simulink model "L4_SIM"  (R2018a)
settings: Solver=ode1  StartTime=0.0  StopTime=60  FixedStep=GLB_FIXED_STEP_SIZE_CPV  RelTol=1e-3  EnableMultiTasking=on
undefined symbols (not defined in the file or in its folder): Cf, Chassis, Cr, CYCLE_ACC1_2A__AdaptiveCruiseCtrlMode, CYCLE_ACC1_2A__AdaptiveCruiseCtrlSetSpeed, CYCLE_CCVS1_00__CruiseCtrlSetSpeed, CYCLE_CCVS1_00__WheelBasedVehicleSpeed, CYCLE_EEC1_00__EngSpeed, CYCLE_ETC1_00__TransDrivelineEngaged, CYCLE_ETC2_00__TransActualGearRatio, CYCLE_ETC7_03__TransMode1Indicator, CYCLE_GPS_Latitude, CYCLE_GPS_Longitude, CYCLE_LFE1_00__EngFuelRate, CYCLE_Net_Engine_Percent_Torque, CYCLE_SSI2_03__PitchAngleExRange, CYCLE_TIME, CYCLE_UTM_Origin_X, CYCLE_UTM_Origin_Y, CYCLE_Vehicle_Distance, DiscIntNeverNeededParam, ENUM_J1939_PCC_STATE_T, ENUM_J1939_SWITCH_T, ENUM_STEERING_WHEEL_ANGLE_SENSOR_TYPE_T, GLB_FIXED_STEP_SIZE_CPV, GLB_TRANS_LOSS_TRQ_GEAR_STEP_MPV, GLB_TRANS_LOSS_TRQ_SPD_STEP_MPV, GLB_TRANS_LOSS_TRQ_TABLE_DATA_MPV, GLB_TRANS_LOSS_TRQ_TRQ_STEP_MPV, GLB_VEHICLE_CONFIG_ACCEL_PED_GATEWAY_APV, heading_0, Iz, L4_Controller, lf, lr, position_0, ptc_matlab_lib, STEERCTRL_10ms, SUB_ECU_L4_MABX, SUB_L4_Task_10ms, SUB_L4_Task_10ms_SUB_STEERCTRL, SUB_PLANT_Chassis, Task_10ms, Vx_0
libraries: EmE_MBD_Blockset x81, PTC_MBDS_LIB x71, simulink x38, simulink_extras x1, SUB_L4_Task_10000ms x1, SUB_L4_Task_1000ms x1, SUB_L4_Task_100ms x1, SUB_L4_Task_10ms_SUB_APTC x1, SUB_L4_Task_10ms_SUB_BRKPEDARB x1, SUB_L4_Task_10ms_SUB_FAULT_MANAGER x1, SUB_L4_Task_10ms_SUB_STATE_CONTROL x1, simulink_need_slupdate x1
(part 1 of 6)
settings Model: PauseTimes=1555  Creator=Sundeep.Tuteja  LastModifiedBy=Gennaro.Kukonu
settings SolverCC: AutoInsertRateTranBlk=on
settings OptimizationCC: DefaultUnderspecifiedDataType=single  LifeSpan=inf
settings DebuggingCC: SignalRangeChecking=error  AlgebraicLoopMsg=error  BlockPriorityViolationMsg=error  MinStepSizeMsg=error  TasksWithSamePriorityMsg=error  ParameterDowncastMsg=warning  UnderSpecifiedDataTypeMsg=warning  UnnecessaryDatatypeConvMsg=warning  SignalLabelMismatchMsg=warning  UnconnectedInputMsg=error  UniqueDataStoreMsg=error  BusObjectLabelMismatch=error  StateNameClashWarn=warning  SFExecutionAtInitializationDiag=none
settings CodeAppCC: StateflowObjectComments=on

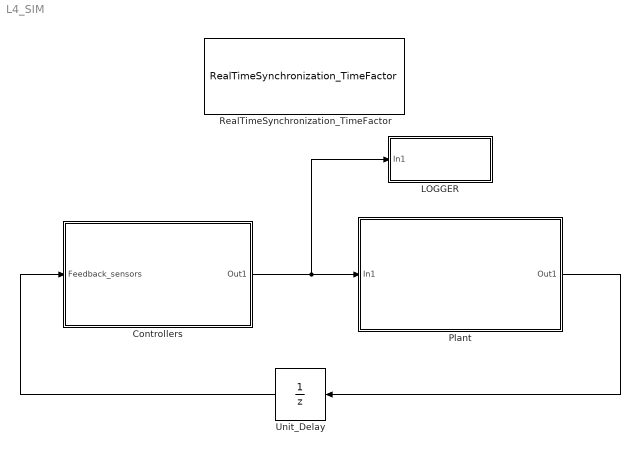
== system L4_SIM ==
  Controllers : Subsystem
  LOGGER : Subsystem
  Plant : Subsystem
      mask Display: image(fullfile(fileparts(which(bdroot(gcs))), '..', 'images', 'truckicon.jpg'));
  RealTimeSynchronization_TimeFactor : PTC_MBDS_LIB/Extras/HMI/RealTimeSynchronization_TimeFactor  Enable=off  TimeFactor=1  TimeFactor_prev=1  PTC_MBDS_BlockVersion=5.41  PTC_BlockType=PTC_MBDS_RealTimeSynchronization_TimeFactor
      settings: SourceProductName=PACCAR Technical Center MBDS Library
  Unit_Delay : UnitDelay  SampleTime=-1
      settings: AttributesFormatString=Init = %<InitialCondition>
  wires:
  Controllers/1(Out1) -> LOGGER/1(In1), Plant/1(In1)
  Plant/1(Out1) -> Unit_Delay/1
  Unit_Delay/1 -> Controllers/1(Feedback_sensors)

== system L4_SIM/Controllers ==
  Feedback_sensors : Inport
  Bus Creator : BusCreator  Inputs=5
  Drive_Cycle : Subsystem
  Operator : Subsystem
  Virtual_Controllers : Subsystem
  Out1 : Outport
  wires:
  Feedback_sensors/1 -> Drive_Cycle/1(Feedback_in)  "Feedback_sensors"
  Drive_Cycle/1(Cycle_out) -> Operator/1(Cycle_in)
  Drive_Cycle/2(Feedback_sensors_out) -> Operator/2(Feedback_sensors_in)
  Operator/1(Cycle_out) -> Virtual_Controllers/1(Cycle_in)
  Operator/2(Feedback_sensors_out) -> Virtual_Controllers/2(Feedback_sensors_in)
  Operator/3(Operator_out) -> Virtual_Controllers/3(Operator_in)
  Virtual_Controllers/1(Cycle_out) -> Bus Creator/1  "Cycle"
  Virtual_Controllers/2(Feedback_sensors_out) -> Bus Creator/2  "Feedback"
  Virtual_Controllers/3(Operator_out) -> Bus Creator/3  "Operator"
  Virtual_Controllers/4(Controller_out) -> Bus Creator/4  "Controller"
  Bus Creator/1 -> Out1/1
  Virtual_Controllers/5(Interfaces_out) -> Bus Creator/5  "Interface"

== system L4_SIM/LOGGER ==
  In1 : Inport
  Bus Creator : BusCreator  Inputs=14
  Bus Creator1 : BusCreator  Inputs=12
  Bus Selector : BusSelector  OutputSignals=Interface.CAN.EEC1_00.SPN513_ActualEngPercTorque,Interface.CAN.EEC1_00.SPN190_EngineSpeed,Interface.CAN.ETC2_00.SPN526_TransActualGearRatio,Interface.CAN.ETC2_00.SPN523_TransCurrentGear,Interface.CAN.EEC3_00.SPN514_NominalFrictionPercTorque,Interface.CAN.CCVS1_00.SPN84_WheelBasedVehicleSpeed,Interface.CAN.CCVS1_00.SPN86_CruiseControlSetSpeed,Interface.CAN.CCVS1_00.SPN527_CruiseControlState,Interface.CAN.EEC2_00.SPN91_AccelPedalPosition1,Interface.CAN.ERC1_0F.SPN520_ActualRetarderPercentTorque,Interface.CAN.ETC1_03.SPN560_TransDrivelineEngaged,Interface.CAN.SSI2_03.SPN4976_PitchAngleExtendedRange,Interface.CAN.CCVS3_00.SPN7319_CruiseControlSpeed,Interface.CAN.VDHR_31.SPN917_TotalVehicleDistanceHiResolution
  Bus Selector1 : BusSelector  OutputSignals=Controller
  Bus Selector2 : BusSelector  OutputSignals=AMT.ShiftControl.Internal.GearNumberCommand,AMT.ShiftControl.Internal.MainClutch,AMT.ShiftControl.Internal.ShiftControlState,AMT.ShiftControl.External.GearNumberActual,AMT.ShiftControl.External.TransStateLock,AMT.ShiftControl.External.TSC1_P32_TE.OCME,AMT.ShiftControl.External.TSC1_P32_TE.TrqReqE,PCI.EngTrqDemand,PCI.EngSpeedRPM,PCI.DriverDemPercentTrq,ABS.FrontAxleSpd,L4_MABX.10msTask.APTC.APTC_arb_pedal_position
  SignalConversion{,1..25} (26 alike) : SignalConversion  ConversionOutput=Contiguous copy  OverrideOpt=off
  Terminator : Terminator
      settings: InitFcn=|
      | try
      |    MBDS_BlockCallback('Update', gcb);
      | end
  Terminator1 : Terminator
      settings: InitFcn=|
      | try
      |    MBDS_BlockCallback('Update', gcb);
      | end
  wires:
  In1/1 -> Bus Selector1/1, Bus Selector/1
  Bus Creator/1 -> Terminator/1
  Bus Selector1/1 -> Bus Selector2/1  "<Controller>"
  Bus Creator1/1 -> Terminator1/1
  Bus Selector/1 -> SignalConversion/1  "<SPN513_ActualEngPercTorque>"
  SignalConversion/1 -> Bus Creator/1  "SPN513_ActualEngPercTorque"
  Bus Selector/2 -> SignalConversion1/1  "<SPN190_EngineSpeed>"
  SignalConversion1/1 -> Bus Creator/2  "SPN190_EngineSpeed"
  Bus Selector/3 -> SignalConversion2/1  "<SPN526_TransActualGearRatio>"
  SignalConversion2/1 -> Bus Creator/3  "SPN526_TransActualGearRatio"
  Bus Selector/4 -> SignalConversion3/1  "<SPN523_TransCurrentGear>"
  SignalConversion3/1 -> Bus Creator/4  "SPN523_TransCurrentGear"
  Bus Selector/5 -> SignalConversion4/1  "<SPN514_NominalFrictionPercTorque>"
  SignalConversion4/1 -> Bus Creator/5  "SPN514_NominalFrictionPercTorque"
  Bus Selector/6 -> SignalConversion5/1  "<SPN84_WheelBasedVehicleSpeed>"
  SignalConversion5/1 -> Bus Creator/6  "SPN84_WheelBasedVehicleSpeed"
  Bus Selector/7 -> SignalConversion6/1  "<SPN86_CruiseControlSetSpeed>"
  SignalConversion6/1 -> Bus Creator/7  "SPN86_CruiseControlSetSpeed"
  Bus Selector/8 -> SignalConversion7/1  "<SPN527_CruiseControlState>"
  SignalConversion7/1 -> Bus Creator/8  "SPN527_CruiseControlState"
  Bus Selector/9 -> SignalConversion8/1  "<SPN91_AccelPedalPosition1>"
  SignalConversion8/1 -> Bus Creator/9  "SPN91_AccelPedalPosition1"
  Bus Selector/10 -> SignalConversion9/1  "<SPN520_ActualRetarderPercentTorque>"
  SignalConversion9/1 -> Bus Creator/10  "SPN520_ActualRetarderPercentTorque"
  Bus Selector/11 -> SignalConversion10/1  "<SPN560_TransDrivelineEngaged>"
  SignalConversion10/1 -> Bus Creator/11  "SPN560_TransDrivelineEngaged"
  Bus Selector/12 -> SignalConversion11/1  "<SPN4976_PitchAngleExtendedRange>"
  SignalConversion11/1 -> Bus Creator/12  "SPN4976_PitchAngleExtendedRange"
  Bus Selector/13 -> SignalConversion12/1  "<SPN7319_CruiseControlSpeed>"
  SignalConversion12/1 -> Bus Creator/13  "SPN7319_CruiseControlSpeed"
  Bus Selector/14 -> SignalConversion13/1  "<SPN917_TotalVehicleDistanceHiResolution>"
  SignalConversion13/1 -> Bus Creator/14  "SPN917_TotalVehicleDistanceHiResolution"
  Bus Selector2/11 -> SignalConversion14/1  "<FrontAxleSpd>"
  SignalConversion14/1 -> Bus Creator1/11  "FrontAxleSpd"
  Bus Selector2/10 -> SignalConversion15/1  "<DriverDemPercentTrq>"
  SignalConversion15/1 -> Bus Creator1/10  "DriverDemPercentTrq"
  Bus Selector2/9 -> SignalConversion16/1  "<EngSpeedRPM>"
  SignalConversion16/1 -> Bus Creator1/9  "EngSpeedRPM"
  Bus Selector2/8 -> SignalConversion17/1  "<EngTrqDemand>"
  SignalConversion17/1 -> Bus Creator1/8  "EngTrqDemand"
  Bus Selector2/7 -> SignalConversion18/1  "<TrqReqE>"
  SignalConversion18/1 -> Bus Creator1/7  "TrqReq"
  Bus Selector2/6 -> SignalConversion19/1  "<OCME>"
  SignalConversion19/1 -> Bus Creator1/6  "OCM"
  Bus Selector2/5 -> SignalConversion20/1  "<TransStateLock>"
  SignalConversion20/1 -> Bus Creator1/5  "TransStateLock"
  Bus Selector2/4 -> SignalConversion21/1  "<GearNumberActual>"
  SignalConversion21/1 -> Bus Creator1/4  "GearNumberActual"
  Bus Selector2/3 -> SignalConversion22/1  "<ShiftControlState>"
  SignalConversion22/1 -> Bus Creator1/3  "ShiftControlState"
  Bus Selector2/2 -> SignalConversion23/1  "<MainClutch>"
  SignalConversion23/1 -> Bus Creator1/2  "MainClutch"
  Bus Selector2/1 -> SignalConversion24/1  "<GearNumberCommand>"
  SignalConversion24/1 -> Bus Creator1/1  "GearNumberCommand"
  Bus Selector2/12 -> SignalConversion25/1  "<APTC_arb_pedal_position>"
  SignalConversion25/1 -> Bus Creator1/12  "AcceleratorPedalPosOut"

== system L4_SIM/Plant ==
  In1 : Inport
  Bus Creator : BusCreator  Inputs=3
  Bus Selector : BusSelector  OutputSignals=Feedback,Operator,Cycle,Controller
  PlantModel : Subsystem
  Out1 : Outport
  wires:
  In1/1 -> Bus Selector/1
  Bus Selector/3 -> PlantModel/3(Cycle)  "<Cycle>"
  Bus Selector/2 -> PlantModel/2(Driver)  "<Operator>"
  Bus Selector/4 -> PlantModel/4(Control)  "<Controller>"
  PlantModel/2(Engine_O) -> Bus Creator/2  "Engine"
  PlantModel/1(Chassis_O) -> Bus Creator/1  "Chassis"
  Bus Creator/1 -> Out1/1
  Bus Selector/1 -> PlantModel/1(FB)  "<Feedback>"
  PlantModel/3(Nav_O) -> Bus Creator/3  "Navigation"

== system L4_SIM/Controllers/Drive_Cycle ==
  Feedback_in : Inport
  Bias : Bias  Bias=-1
  Bus Selector1 : BusSelector  OutputSignals=ActualVehicleDistance
  Bus Selector2 : BusSelector  OutputSignals=Chassis.MeasuredVehicleSpeed_kph
  Constant1 : PTC_MBDS_LIB/Extras/Sources/Constant  Value2=1/3.6  PTC_MBDS_BlockVersion=5.41  PTC_BlockType=PTC_MBDS_Constant
      settings: SourceProductName=PACCAR Technical Center MBDS Library
  Constant3 : PTC_MBDS_LIB/Extras/Sources/Constant  Value2=CYCLE_Vehicle_Distance  PTC_MBDS_BlockVersion=5.41  PTC_BlockType=PTC_MBDS_Constant
      settings: SourceProductName=PACCAR Technical Center MBDS Library
      settings: AttributesFormatString=|
      | Value: <16520 X 1>
      | Unit: 'm'
  DriveCycle : Subsystem
  GE : PTC_MBDS_LIB/MBDS Standard Library/Basic Operations/Logic and Bit Operations/GE  InputSameDT=on  PTC_MBDS_BlockVersion=5.41  PTC_BlockType=PTC_MBDS_GE
      settings: SourceProductName=PACCAR Technical Center MBDS Library
  Product : Product  Inputs=**  OutDataTypeStr=Inherit: Inherit via back propagation  SaturateOnIntegerOverflow=on  InputSameDT=on
      settings: AttributesFormatString=Saturate: %<SaturateOnIntegerOverflow>
  Selector2 : Selector  IndexOptions=Index vector (port)  Indices=[1 3]  OutputSizes=1
  Stop Simulation : Stop
  Width1 : Width  DataType=uint32
  Cycle_out : Outport
  Feedback_sensors_out : Outport  Port=2
  wires:
  Feedback_in/1 -> Feedback_sensors_out/1, Bus Selector2/1
  Constant1/1 -> Product/2
  Product/1 -> DriveCycle/1(MeasuredVehicleSpeed_mps)  "MeasuredVehicleSpeed_mps"
  Bus Selector2/1 -> Product/1  "<MeasuredVehicleSpeed_kph>"
  DriveCycle/1(Cycle_out) -> Bus Selector1/1, Cycle_out/1  "Cycle"
  Selector2/1 -> Bias/1
  Width1/1 -> Selector2/2
  Constant3/1 -> Selector2/1, Width1/1  "CYCLE_Vehicle_Distance"
  Bus Selector1/1 -> GE/1  "<ActualVehicleDistance>"
  GE/1 -> Stop Simulation/1
  Bias/1 -> GE/2

== system L4_SIM/Controllers/Operator ==
  Cycle_in : Inport
  Feedback_sensors_in : Inport  Port=2
  Bus Creator : BusCreator  Inputs=4
  Bus Selector : BusSelector  OutputSignals=RefVehSpeed,RefVehPosition,CCSetSpeed,L4OperatorEnable
  Bus Selector1 : BusSelector  OutputSignals=Chassis.MeasuredVehicleSpeed_kph,Navigation.VehPosition
  Subsystem : Subsystem
  Cycle_out : Outport
  Feedback_sensors_out : Outport  Port=2
  Operator_out : Outport  Port=3
  wires:
  Cycle_in/1 -> Cycle_out/1, Bus Selector/1  "Cycle"
  Feedback_sensors_in/1 -> Bus Selector1/1, Feedback_sensors_out/1  "Feedback_sensors"
  Bus Selector/1 -> Subsystem/1(RefVehSpeed[km/h])  "<RefVehSpeed>"
  Bus Selector/3 -> Subsystem/3(CCSetSpeed[km/h])  "<CCSetSpeed>"
  Bus Selector1/1 -> Subsystem/5(MeasuredVehicleSpeed[km/h])  "<MeasuredVehicleSpeed_kph>"
  Subsystem/1(BrkDrv[0-1]) -> Bus Creator/1
  Subsystem/2(PedDrv[0-1]) -> Bus Creator/2
  Bus Creator/1 -> Operator_out/1  "Operator"
  Subsystem/3(OperatorEnable) -> Bus Creator/3  "OperatorEnable"
  Bus Selector/4 -> Subsystem/4(OperatorEnableCycle)  "<L4OperatorEnable>"
  Bus Selector/2 -> Subsystem/2(RefVehPosition[m])  "<RefVehPosition>"
  Subsystem/4(TargetHeading) -> Bus Creator/4  "TargetHeading"
  Bus Selector1/2 -> Subsystem/6(MeasuredVehiclePosition[m])  "<VehPosition>"

== system L4_SIM/Controllers/Virtual_Controllers ==
  Cycle_in : Inport
  Feedback_sensors_in : Inport  Port=2
  Operator_in : Inport  Port=3
  ABS : Subsystem
  Bus Creator1 : BusCreator  Inputs=4
  Bus Creator2 : BusCreator  Inputs=9
  ERAD : Subsystem
  Interface_Abstraction : Subsystem
  L4_MABX : Subsystem
  PACC : Subsystem
  PCC : Subsystem
  PCI : Subsystem
  TCM : Subsystem
  Unit_Delay : UnitDelay  SampleTime=-1
      settings: AttributesFormatString=Init = %<InitialCondition>
  VECU : Subsystem
  VEMC : Subsystem
  Cycle_out : Outport
  Feedback_sensors_out : Outport  Port=2
  Operator_out : Outport  Port=3
  Controller_out : Outport  Port=4
  Interfaces_out : Outport  Port=5
  wires:
  Bus Creator1/1 -> Interface_Abstraction/1(Inport)
  Interface_Abstraction/1(Outport) -> ERAD/1(In1), TCM/1(In1), VEMC/1(In1), VECU/1(In1), PCI/1(In), PCC/1(In1), PACC/1(In1), L4_MABX/1(input), Interfaces_out/1, ABS/1(input)
  Cycle_in/1 -> Cycle_out/1, Bus Creator1/1  "Cycle"
  Feedback_sensors_in/1 -> Bus Creator1/2, Feedback_sensors_out/1  "Feedback_sensors"
  Operator_in/1 -> Bus Creator1/3, Operator_out/1  "Operator"
  TCM/1(Out1) -> Bus Creator2/7  "AMT"
  ABS/1(Out1) -> Bus Creator2/1  "ABS"
  PCI/1(Out1) -> Bus Creator2/6  "PCI"
  PACC/1(Out1) -> Bus Creator2/4  "PACC"
  L4_MABX/1(Out1) -> Bus Creator2/3  "L4_MABX"
  PCC/1(Out1) -> Bus Creator2/5  "PCC"
  Bus Creator2/1 -> Unit_Delay/1, Controller_out/1  "Feedback_controllers"
  ERAD/1(Out1) -> Bus Creator2/2  "ERAD"
  Unit_Delay/1 -> Bus Creator1/4  "Feedback_controllers"
  VECU/1(Out1) -> Bus Creator2/8  "VECU"
  VEMC/1(Out1) -> Bus Creator2/9  "VEMC"

== system L4_SIM/Plant/PlantModel ==
  FB : Inport
  Driver : Inport  Port=2
  Cycle : Inport  Port=3
  Control : Inport  Port=4
  Bus Selector : BusSelector  OutputSignals=BrkDrv
  Bus Selector2 : BusSelector  OutputSignals=PCI,AMT,ABS,L4_MABX
  Chassis : Subsystem  AncestorBlock=SUB_PLANT_Chassis/Chassis
  Engine : SUB_PLANT_Engine/Engine
      link override Bus Selector1: OutputSignals=Chassis.TrqFromClutch,Chassis.ClutchState,Chassis.EngSpdClutchClosed
  Navigation : Subsystem
  Chassis_O : Outport
  Engine_O : Outport  Port=2
  Nav_O : Outport  Port=3
  wires:
  Engine/1 -> Chassis/1(Engine), Engine_O/1
  Driver/1 -> Bus Selector/1
  Bus Selector/1 -> Chassis/2(FoundationBrakes)  "<BrkDrv>"
  Cycle/1 -> Chassis/4(Cycle)
  Control/1 -> Bus Selector2/1
  Bus Selector2/1 -> Engine/2  "<PCI>"
  Bus Selector2/2 -> Chassis/3(AMT)  "<AMT>"
  Bus Selector2/3 -> Chassis/5(ABS)  "<ABS>"
  Chassis/1(ChassisMdl_O) -> Navigation/1(In1), Chassis_O/1
  Bus Selector2/4 -> Chassis/6(L4_MABX)  "<L4_MABX>"
  FB/1 -> Chassis/7(Navigation), Engine/1
  Navigation/1(Out1) -> Nav_O/1  "Navigation"

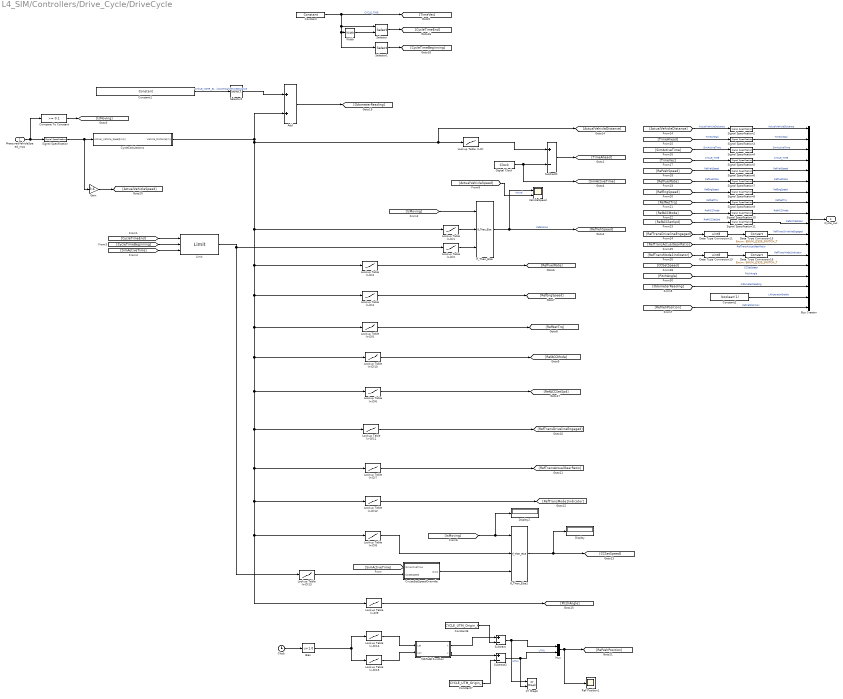
== system L4_SIM/Controllers/Drive_Cycle/DriveCycle ==
  MeasuredVehicleSpeed_mps : Inport
  Add : Sum  OutDataTypeStr=Inherit: Inherit via back propagation  SaturateOnIntegerOverflow=on  InputSameDT=on
      settings: AttributesFormatString=Saturate: %<SaturateOnIntegerOverflow>
  Bias : Bias  Bias=1.0
  Bus Creator : BusCreator  Inputs=18
  Clock : Clock
  Compare To Constant : simulink/Logic and Bit Operations/Compare To Constant  relop=>=  const=0.1  OutDataTypeStr=boolean
  Constant : PTC_MBDS_LIB/Extras/Sources/Constant  Value2=CYCLE_TIME  PTC_MBDS_BlockVersion=5.41  PTC_BlockType=PTC_MBDS_Constant
      settings: SourceProductName=PACCAR Technical Center MBDS Library
      settings: AttributesFormatString=|
      | Value: <16520 X 1>
      | Unit: 's'
  Constant1 : PTC_MBDS_LIB/Extras/Sources/Constant  Value2=CYCLE_VDHR_31__HghRslutionTotalVehicleDistance  PTC_MBDS_BlockVersion=5.41  PTC_BlockType=PTC_MBDS_Constant
      settings: SourceProductName=PACCAR Technical Center MBDS Library
      settings: AttributesFormatString=|
      | Value: <16520 X 1>
      | Unit: 'm'
  Constant2 : Constant  Value=boolean(1)
  Constant6 : Constant  Value=CYCLE_UTM_Origin_X
  Constant7 : Constant  Value=CYCLE_UTM_Origin_Y
  CruiseSetSpeedOverride : Subsystem
  CycleCalculations : Subsystem
  Data Type Conversion11 : DataTypeConversion  OutDataTypeStr=uint8  SaturateOnIntegerOverflow=on
  Data Type Conversion13 : DataTypeConversion  OutDataTypeStr=uint8  SaturateOnIntegerOverflow=on
  Data Type Conversion15 : DataTypeConversion  OutDataTypeStr=Enum: ENUM_J1939_SWITCH_T  SaturateOnIntegerOverflow=on
  Data Type Conversion16 : DataTypeConversion  OutDataTypeStr=Enum: ENUM_J1939_SWITCH_T  SaturateOnIntegerOverflow=on
  Digital Clock : DigitalClock  SampleTime=GLB_FIXED_STEP_SIZE_CPV
  Display : Display
  Display2 : Display
  Gain : Gain  Gain=3.6
  If_Then_Else : PTC_MBDS_LIB/Extras/Signal Routing/If_Then_Else  PTC_MBDS_BlockVersion=5.41  PTC_BlockType=PTC_MBDS_If_Then_Else
      settings: SourceProductName=PACCAR Technical Center MBDS Library
  If_Then_Else1 : PTC_MBDS_LIB/Extras/Signal Routing/If_Then_Else  PTC_MBDS_BlockVersion=5.41  PTC_BlockType=PTC_MBDS_If_Then_Else
      settings: SourceProductName=PACCAR Technical Center MBDS Library
  Limit : PTC_MBDS_LIB/MBDS Standard Library/Basic Operations/Non-Linear Operations/Limit  MXMN_Enabled=on  MX=0  MN=0  B_min_Enabled=off  B_max_Enabled=off  OutDataTypeStr=Inherit: Inherit via back propagation  SaturateOnIntegerOverflow=on  InputSameDT=on  InOutSameDT=on  PTC_MBDS_BlockVersion=5.41  PTC_BlockType=PTC_MBDS_Limit
      settings: AttributesFormatString=Saturate: on  SourceProductName=PACCAR Technical Center MBDS Library
  Lookup Table (n-D) : Lookup_n-D  NumberOfTableDimensions=1  BreakpointsForDimension1=CYCLE_Vehicle_Distance  Table=CYCLE_TIME  ExtrapMethod=Clip  DiagnosticForOutOfRangeInput=Error  InputSameDT=on
  Lookup Table (n-D)1 : Lookup_n-D  NumberOfTableDimensions=1  BreakpointsForDimension1=CYCLE_Vehicle_Distance  Table=CYCLE_CCVS1_00__WheelBasedVehicleSpeed  ExtrapMethod=Clip  DiagnosticForOutOfRangeInput=Error  InputSameDT=on
  Lookup Table (n-D)10 : Lookup_n-D  NumberOfTableDimensions=1  BreakpointsForDimension1=CYCLE_Vehicle_Distance  Table=CYCLE_ACC1_2A__AdaptiveCruiseCtrlMode  InterpMethod=Flat  ExtrapMethod=Clip  DiagnosticForOutOfRangeInput=Error  InputSameDT=on
  Lookup Table (n-D)11 : Lookup_n-D  NumberOfTableDimensions=1  BreakpointsForDimension1=CYCLE_Vehicle_Distance  Table=CYCLE_ETC1_00__TransDrivelineEngaged  InterpMethod=Flat  ExtrapMethod=Clip  DiagnosticForOutOfRangeInput=Error  InputSameDT=on
  Lookup Table (n-D)12 : Lookup_n-D  NumberOfTableDimensions=1  BreakpointsForDimension1=CYCLE_Vehicle_Distance  Table=CYCLE_ETC7_03__TransMode1Indicator  InterpMethod=Flat  ExtrapMethod=Clip  DiagnosticForOutOfRangeInput=Error  InputSameDT=on
  Lookup Table (n-D)13 : Lookup_n-D  NumberOfTableDimensions=1  BreakpointsForDimension1=CYCLE_TIME  Table=CYCLE_CCVS1_00__CruiseCtrlSetSpeed  ExtrapMethod=Clip  DiagnosticForOutOfRangeInput=Error  InputSameDT=on
  Lookup Table (n-D)14 : Lookup_n-D  NumberOfTableDimensions=1  BreakpointsForDimension1=CYCLE_TIME  Table=CYCLE_GPS_Latitude  ExtrapMethod=Clip  DiagnosticForOutOfRangeInput=Error  InputSameDT=on
  Lookup Table (n-D)15 : Lookup_n-D  NumberOfTableDimensions=1  BreakpointsForDimension1=CYCLE_TIME  Table=CYCLE_GPS_Longitude  ExtrapMethod=Clip  DiagnosticForOutOfRangeInput=Error  InputSameDT=on
  Lookup Table (n-D)2 : Lookup_n-D  NumberOfTableDimensions=1  BreakpointsForDimension1=CYCLE_TIME  Table=CYCLE_CCVS1_00__WheelBasedVehicleSpeed  ExtrapMethod=Clip  DiagnosticForOutOfRangeInput=Error  InputSameDT=on
  Lookup Table (n-D)3 : Lookup_n-D  NumberOfTableDimensions=1  BreakpointsForDimension1=CYCLE_Vehicle_Distance  Table=CYCLE_LFE1_00__EngFuelRate  ExtrapMethod=Clip  DiagnosticForOutOfRangeInput=Error  InputSameDT=on
  Lookup Table (n-D)4 : Lookup_n-D  NumberOfTableDimensions=1  BreakpointsForDimension1=CYCLE_Vehicle_Distance  Table=CYCLE_EEC1_00__EngSpeed  ExtrapMethod=Clip  DiagnosticForOutOfRangeInput=Error  InputSameDT=on
  Lookup Table (n-D)5 : Lookup_n-D  NumberOfTableDimensions=1  BreakpointsForDimension1=CYCLE_Vehicle_Distance  Table=CYCLE_Net_Engine_Percent_Torque  ExtrapMethod=Clip  DiagnosticForOutOfRangeInput=Error  InputSameDT=on
  Lookup Table (n-D)6 : Lookup_n-D  NumberOfTableDimensions=1  BreakpointsForDimension1=CYCLE_Vehicle_Distance  Table=CYCLE_ACC1_2A__AdaptiveCruiseCtrlSetSpeed  ExtrapMethod=Clip  DiagnosticForOutOfRangeInput=Error  InputSameDT=on
  Lookup Table (n-D)7 : Lookup_n-D  NumberOfTableDimensions=1  BreakpointsForDimension1=CYCLE_Vehicle_Distance  Table=CYCLE_ETC2_00__TransActualGearRatio  ExtrapMethod=Clip  DiagnosticForOutOfRangeInput=Error  InputSameDT=on
  Lookup Table (n-D)8 : Lookup_n-D  NumberOfTableDimensions=1  BreakpointsForDimension1=CYCLE_Vehicle_Distance  Table=CYCLE_CCVS1_00__CruiseCtrlSetSpeed  ExtrapMethod=Clip  DiagnosticForOutOfRangeInput=Error  InputSameDT=on
  Lookup Table (n-D)9 : Lookup_n-D  NumberOfTableDimensions=1  BreakpointsForDimension1=CYCLE_Vehicle_Distance  Table=CYCLE_SSI2_03__PitchAngleExRange  ExtrapMethod=Clip  DiagnosticForOutOfRangeInput=Error  InputSameDT=on
  MATLAB Function : MATLAB Function  TreatAsAtomicUnit=on
  Mux : Mux  Inputs=2
  Ref Position1 : Scope
  Selector : Selector  IndexOptions=Index vector (port)  Indices=[1 3]  OutputSizes=1
  Selector1 : Selector  IndexOptions=Index vector (dialog)  Indices=1  OutputSizes=1
  Selector2 : Selector  IndexOptions=Index vector (dialog)  Indices=1  OutputSizes=1
  Signal Specification{,2..11} (11 alike) : SignalSpecification  OutDataTypeStr=double
  Subtract : Sum  Inputs=+-
  Subtract1 : Sum  Inputs=+-  OutDataTypeStr=Inherit: Inherit via back propagation  SaturateOnIntegerOverflow=on  InputSameDT=on
      settings: AttributesFormatString=Saturate: %<SaturateOnIntegerOverflow>
  Subtract2 : Sum  Inputs=+-
  VehicleSpeed : Scope  NumInputPorts=2
  Width : Width  DataType=uint32
  XY Graph : simulink/Sinks/XY Graph  xmin=-100  xmax=100  ymin=-100  ymax=100  st=-1
  Cycle_out : Outport
  wires:
  MeasuredVehicleSpeed_mps/1 -> Signal Specification/1, Compare To Constant/1
  Lookup Table (n-D)/1 -> Subtract1/1
  Digital Clock/1 -> [SimActiveTime], Subtract1/2
  Subtract1/1 -> [TimeAhead]
  Compare To Constant/1 -> [IsMoving]
  [IsMoving] -> If_Then_Else/1
  Lookup Table (n-D)2/1 -> If_Then_Else/3
  Lookup Table (n-D)3/1 -> [RefFuelRate]
  Lookup Table (n-D)5/1 -> [RefNetTrq]
  Lookup Table (n-D)10/1 -> [RefACCMode]
  [RefTransDrivelineEngaged] -> Data Type Conversion11/1
  [RefTransMode1Indicator] -> Data Type Conversion13/1
  Bus Creator/1 -> Cycle_out/1
  [ActualVehicleDistance] -> Signal Specification2/1  "ActualVehicleDistance"
  [TimeAhead] -> Signal Specification3/1  "TimeAhead"
  [SimActiveTime] -> Signal Specification4/1  "SimActiveTime"
  [TimeVec] -> Signal Specification5/1  "CYCLE_TIME"
  [RefVehSpeed] -> Signal Specification6/1  "RefVehSpeed"
  [RefFuelRate] -> Signal Specification7/1  "RefFuelRate"
  [RefEngSpeed] -> Signal Specification8/1  "RefEngSpeed"
  [RefNetTrq] -> Signal Specification9/1  "RefNetTrq"
  [RefACCSetSpd] -> Signal Specification11/1  "RefACCSetSpd"
  Data Type Conversion11/1 -> Data Type Conversion15/1
  Data Type Conversion13/1 -> Data Type Conversion16/1
  [RefACCMode] -> Signal Specification10/1  "RefACCMode"
  Lookup Table (n-D)1/1 -> If_Then_Else/2
  Lookup Table (n-D)4/1 -> [RefEngSpeed]
  Lookup Table (n-D)6/1 -> [RefACCSetSpd]
  Lookup Table (n-D)11/1 -> [RefTransDrivelineEngaged]
  Lookup Table (n-D)7/1 -> [RefTransActualGearRatio]
  Lookup Table (n-D)12/1 -> [RefTransMode1Indicator]
  Lookup Table (n-D)9/1 -> [PitchAngle]
  Lookup Table (n-D)8/1 -> If_Then_Else1/2
  [SimActiveTime] -> CruiseSetSpeedOverride/1(SimActiveTime)
  [SimActiveTime] -> Limit/3
  Constant/1 -> [TimeVec], Selector1/1, Width/1, Selector/1  "CYCLE_TIME"
  Width/1 -> Selector/2
  Selector/1 -> [CycleTimeEnd]
  [CycleTimeEnd] -> Limit/1
  Selector1/1 -> [CycleTimeBeginning]
  [CycleTimeBeginning] -> Limit/2
  Constant1/1 -> Selector2/1  "CYCLE_VDHR_31__HghRslutionTotalVehicleDistance"
  Add/1 -> [OdometerReading]
  Selector2/1 -> Add/1
  Data Type Conversion15/1 -> Bus Creator/11  "RefTransDrivelineEngaged"
  Data Type Conversion16/1 -> Bus Creator/13  "RefTransMode1Indicator"
  Signal Specification2/1 -> Bus Creator/1  "ActualVehicleDistance"
  Signal Specification3/1 -> Bus Creator/2  "TimeAhead"
  Signal Specification4/1 -> Bus Creator/3  "SimActiveTime"
  Signal Specification5/1 -> Bus Creator/4  "CYCLE_TIME"
  Signal Specification6/1 -> Bus Creator/5  "RefVehSpeed"
  Signal Specification7/1 -> Bus Creator/6  "RefFuelRate"
  Signal Specification8/1 -> Bus Creator/7  "RefEngSpeed"
  Signal Specification9/1 -> Bus Creator/8  "RefNetTrq"
  Signal Specification10/1 -> Bus Creator/9  "RefACCMode"
  Signal Specification11/1 -> Bus Creator/10  "RefACCSetSpd"
  [RefTransActualGearRatio] -> Bus Creator/12  "RefTransActualGearRatio"
  [CCSetSpeed] -> Bus Creator/14  "CCSetSpeed"
  [PitchAngle] -> Bus Creator/15  "PitchAngle"
  [OdometerReading] -> Bus Creator/16  "OdometerReading"
  Limit/1 -> Lookup Table (n-D)13/1, Lookup Table (n-D)2/1
  If_Then_Else1/1 -> Display/1, [CCSetSpeed]
  [IsMoving] -> Display2/1, If_Then_Else1/1
  CruiseSetSpeedOverride/1(Out1) -> If_Then_Else1/3
  Lookup Table (n-D)13/1 -> CruiseSetSpeedOverride/2(CCSetSpeed)
  Constant2/1 -> Bus Creator/17  "L4OperatorEnable"
  Constant6/1 -> Subtract/2
  CycleCalculations/1(Vehicle_Distance[m]) -> Lookup Table (n-D)/1, [ActualVehicleDistance], Lookup Table (n-D)9/1, Lookup Table (n-D)8/1, Lookup Table (n-D)12/1, Lookup Table (n-D)7/1, Lookup Table (n-D)11/1, Lookup Table (n-D)6/1, Lookup Table (n-D)10/1, Lookup Table (n-D)5/1, Lookup Table (n-D)4/1, Lookup Table (n-D)3/1, Lookup Table (n-D)1/1, Add/2
  MATLAB Function/1(x) -> Subtract/1
  Lookup Table (n-D)14/1 -> MATLAB Function/1(Lat)
  Lookup Table (n-D)15/1 -> MATLAB Function/2(Lon)
  MATLAB Function/2(y) -> Subtract2/1
  Constant7/1 -> Subtract2/2
  If_Then_Else/1 -> VehicleSpeed/1, [RefVehSpeed]  "Reference"
  [ActualVehicleSpeed] -> VehicleSpeed/2  "Actual"
  Signal Specification/1 -> Gain/1, CycleCalculations/1(Actual_Vehicle_Speed[m/s])
  Gain/1 -> [ActualVehicleSpeed]
  Subtract2/1 -> XY Graph/2, Mux/2  "UTMy"
  Subtract/1 -> XY Graph/1, Mux/1  "UTMx"
  Bias/1 -> Lookup Table (n-D)15/1, Lookup Table (n-D)14/1
  Clock/1 -> Bias/1
  Mux/1 -> Ref Position1/1, [RefVehPosition]
  [RefVehPosition] -> Bus Creator/18  "RefVehPosition"

== system L4_SIM/Controllers/Operator/Subsystem ==
  note: Gains Added in own block
      | so they can be changed in
      | ICR_init.m file.  Acc and Brk
      | Gains should be equal, or it
      | will cause dynamic issues (PID
      | for Acc and Brk are exactly the
      | same, making different gains
      | between the pedals will cause
      | the model to behave differently).
      | This is applicable for the dyno.
  RefVehSpeed[km/h] : Inport  Unit=km/h
  RefVehPosition[m] : Inport  Port=2  Unit=km/h
  CCSetSpeed[km/h] : Inport  Port=3  Unit=km/h
  OperatorEnableCycle : Inport  Port=4  Unit=km/h
  MeasuredVehicleSpeed[km/h] : Inport  Port=5  Unit=km/h
  MeasuredVehiclePosition[m] : Inport  Port=6  Unit=km/h
  Gains : Subsystem
  HeadingController : Subsystem
  PedalArbitration : Subsystem
  SpdControlBrake : Subsystem
  SpdControlTraction : Subsystem
  Unit Delay : UnitDelay  InitialCondition=true  SampleTime=-1
  Unit Delay1 : UnitDelay  InitialCondition=true  SampleTime=-1
  BrkDrv[0-1] : Outport
  PedDrv[0-1] : Outport  Port=2
  OperatorEnable : Outport  Port=3
  TargetHeading : Outport  Port=4
  wires:
  PedalArbitration/1(BrkDrv) -> BrkDrv[0-1]/1  "BrkDrv"
  [VehSpdKph] -> PedalArbitration/3(VehSpdAct)
  [EngSpdGovReset] -> Unit Delay/1
  [VehSpdKph] -> SpdControlBrake/2(VehSpdAct)
  Unit Delay1/1 -> SpdControlBrake/4(Reset)
  PedalArbitration/2(PedDrv) -> PedDrv[0-1]/1  "PedDrv"
  [Gains_Brk] -> SpdControlBrake/3(Gains)
  MeasuredVehicleSpeed[km/h]/1 -> [VehSpdKph]
  PedalArbitration/3(EngSpdGovReset) -> [EngSpdGovReset]
  [VehSpdKph] -> SpdControlTraction/2(VehSpdAct)
  SpdControlTraction/1(PedalComGov(0-1)) -> PedalArbitration/1(PedGov)
  [VehSpdTarget] -> SpdControlBrake/1(VehSpdTarget)
  [BrkSpdGovReset] -> Unit Delay1/1
  [VehSpdTarget] -> PedalArbitration/4(VehSpdTarget)
  SpdControlBrake/1(BrakeComGov(0-1)) -> PedalArbitration/2(BrkGov)
  Unit Delay/1 -> SpdControlTraction/4(Reset)
  PedalArbitration/4(BrakeSpdGovReset) -> [BrkSpdGovReset]
  CCSetSpeed[km/h]/1 -> [CCSetSpd]
  [CCSetSpd] -> PedalArbitration/5(CCSetSpd)
  [VehSpdTarget] -> SpdControlTraction/1(VehSpdTarget)
  Gains/1(Gains_Acc) -> SpdControlTraction/3(Gains)
  Gains/2(Gains_Brk) -> [Gains_Brk]
  RefVehSpeed[km/h]/1 -> [VehSpdTarget]
  OperatorEnableCycle/1 -> OperatorEnable/1
  HeadingController/1(TargetHeading) -> TargetHeading/1
  [VehPosTarget] -> HeadingController/2(<Waypoint>)
  [VehPosition] -> HeadingController/1(<VehPosition>)
  RefVehPosition[m]/1 -> [VehPosTarget]
  MeasuredVehiclePosition[m]/1 -> [VehPosition]

== system L4_SIM/Controllers/Virtual_Controllers/ABS ==
  input : Inport
  Add : Sum
  Bus Creator : BusCreator  Inputs=13
  Bus Creator1 : BusCreator  Inputs=2
  Bus Creator2 : BusCreator  Inputs=2
  Bus Selector : BusSelector  OutputSignals=Feedback_sensors.Chassis.AxleSpeeds,Feedback_controllers.L4_MABX.10msTask.SteeringControl.DesSteeringAngle
  Constant : PTC_MBDS_LIB/Extras/Sources/Constant  Value2=ABS_VEHICLE_MASS_APV  PTC_MBDS_BlockVersion=5.41  PTC_BlockType=PTC_MBDS_Constant
      settings: SourceProductName=PACCAR Technical Center MBDS Library
      settings: AttributesFormatString=|
      | Value: 29491
      | Unit: 'kg'
  Constant{1..3,6..9} (7 alike) : Constant  Value=0
  Constant5 : Constant  Value=ENUM_STEERING_WHEEL_ANGLE_SENSOR_TYPE_T.NOT_AVAILABLE
  ConvertRPM2kph : Subsystem
  Demux : Demux
  Gain : Gain  Gain=1/2
  Out1 : Outport
  wires:
  input/1 -> Bus Selector/1
  Constant/1 -> Bus Creator/1  "ABS_VEHICLE_MASS_APV"
  Bus Creator/1 -> Out1/1
  Demux/1 -> [LF_WhlSpd]
  Demux/2 -> [LR_WhlSpd]
  Demux/3 -> [RF_WhlSpd]
  Demux/4 -> [RR_WhlSpd]
  Bus Selector/1 -> ConvertRPM2kph/1(<AxleSpeeds>)  "<AxleSpeeds>"
  ConvertRPM2kph/1(Spd) -> Demux/1
  [LF_WhlSpd] -> Bus Creator/2  "LF_WhlSpd"
  [LR_WhlSpd] -> Bus Creator/3  "LR_WhlSpd"
  [RF_WhlSpd] -> Bus Creator/4  "RF_WhlSpd"
  [RR_WhlSpd] -> Bus Creator/5  "RR_WhlSpd"
  [LF_WhlSpd] -> Add/1
  [RF_WhlSpd] -> Add/2
  Add/1 -> Gain/1
  Gain/1 -> Bus Creator/6  "FrontAxleSpd"
  Bus Creator2/1 -> Bus Creator/7  "TSC1_P32_BE"
  Constant1/1 -> Bus Creator2/1  "OCME"
  Constant2/1 -> Bus Creator2/2  "TrqReqE"
  Constant3/1 -> Bus Creator/9  "YawRate"
  [SteeringWheelAngle] -> Bus Creator/10  "SteeringWheelAngle"
  Constant6/1 -> Bus Creator/11  "SteeringWheelTurnCounter"
  Constant5/1 -> Bus Creator/12  "SteeringWheelAngleSensorType"
  Constant7/1 -> Bus Creator/13  "LateralAcceleration"
  Constant9/1 -> Bus Creator1/2  "TrqReqR"
  Bus Creator1/1 -> Bus Creator/8  "TSC1_P32_BR"
  Constant8/1 -> Bus Creator1/1  "OCMR"
  Bus Selector/2 -> [SteeringWheelAngle]  "<DesSteeringAngle>"

== system L4_SIM/Controllers/Virtual_Controllers/ERAD ==
  In1 : Inport
  Bus Creator1 : BusCreator  Inputs=1
  Bus Creator2 : BusCreator  Inputs=2
  Constant1 : Constant  Value=0
  Constant2 : Constant  Value=0
  Terminator : Terminator
  Out1 : Outport
  wires:
  Constant1/1 -> Bus Creator2/1  "OCM"
  Constant2/1 -> Bus Creator2/2  "TrqReq"
  Bus Creator2/1 -> Bus Creator1/1  "TSC1_P5_ERAD"
  In1/1 -> Terminator/1
  Bus Creator1/1 -> Out1/1

== system L4_SIM/Controllers/Virtual_Controllers/Interface_Abstraction ==
  Inport : Inport
  Bus Creator : BusCreator  Inputs=6
  Bus Selector : BusSelector  OutputSignals=Feedback_sensors,Feedback_controllers,Operator
  CAN : Subsystem
  HW : Subsystem
  PICBus : Subsystem
  Outport : Outport
  wires:
  Inport/1 -> CAN/1(In1), HW/1(Inport), PICBus/1(In), Bus Selector/1
  CAN/1(Out1) -> Bus Creator/1  "CAN"
  HW/1(Out1) -> Bus Creator/2  "DIGIN"
  Bus Creator/1 -> Outport/1
  Bus Selector/1 -> Bus Creator/3  "<Feedback_sensors>"
  Bus Selector/3 -> Bus Creator/5  "<Operator>"
  Bus Selector/2 -> Bus Creator/4  "<Feedback_controllers>"
  PICBus/1(Out) -> Bus Creator/6  "PIC_Bus"

== system L4_SIM/Controllers/Virtual_Controllers/L4_MABX ==
  input : Inport
  Bus Selector : BusSelector  OutputSignals=Operator.OperatorEnable,DIGIN.PedDrv,CAN.CCVS1_31.SPN597_BrakeSwitch,CAN.EBC2_0B.SPN904_FrontAxleSpd,CAN.HRW_0B.SPN1592_FrontAxleLeftWheelSpeed,CAN.HRW_0B.SPN1593_FrontAxleRightWheelSpeed,CAN.EBC1_0B.SPN1121_EBS_BrakeSwitch,CAN.ETC2_03.SPN524_TransSelectedGear,CAN.ETC2_03.SPN523_TransCurrentGear,CAN.ETC2_03.SPN526_TransActualGearRatio,CAN.EEC1_00.SPN513_ActualEngPercTorque,CAN.EEC1_00.SPN4154_ActualEngPercTorqueFractional,CAN.EEC1_00.SPN190_EngineSpeed,CAN.EEC1_00.SPN512_DriverDemandPercentTorque,CAN.EEC3_00.SPN514_NominalFrictionPercTorque,CAN.EEC3_00.SPN2978_EstimatedEngineParasiticLossesPercTrq,CAN.CVW_03.SPN1760_GrossCombinationVehicleWeight,CAN.ACC1_2A.SPN1796_ACC_DistanceAlertSignal,CAN.ACC1_2A.SPN5022_ForwardCollisionWarning,CAN.EC1_00.SPN544_EngineReferenceTrq,CAN.VDC1_0B.SPN1816_ROP_EngineControlActive,CAN.VDC1_0B.SPN1818_ROP_BrakeControlActive,CAN.VDC1_0B.SPN1817_YC_EngineControlActive,CAN.VDC1_0B.SPN1819_YC_BrakeControlActive,CAN.VDC2_0B.SPN1807_SteeringWheelAngle,CAN.VDC2_0B.SPN1808_YawRate,CAN.AMB_00.SPN108_BarometricPressure,CAN.AMB_00.SPN171_AmbientAirTemperature,CAN.PosRapidUpdate_01.Latitude,CAN.PosRapidUpdate_01.Longitude,CAN.GNSSDOP_01.HDOP,CAN.VDC2_0B.SPN1810_LongitudinalAcceleration,CAN.VDC2_0B.SPN1811_SteeringWheelTurnCounter,CAN.VDC2_0B.SPN1812_SteeringWheelAngleSensorType,CAN.VDC2_0B.SPN1809_LateralAcceleration,PIC_Bus
  Constant{,1,3..4} (4 alike) : Constant  Value=0
  Constant2 : Constant  Value=20
  Constant5 : Constant  Value=true
  Ground : Ground  InitFcn=|
      | try
      |    MBDS_BlockCallback('Update', gcb);
      | end
  Ground1 : Ground  InitFcn=|
      | try
      |    MBDS_BlockCallback('Update', gcb);
      | end
  Ground2 : Ground  InitFcn=|
      | try
      |    MBDS_BlockCallback('Update', gcb);
      | end
  Ground3 : Ground  InitFcn=|
      | try
      |    MBDS_BlockCallback('Update', gcb);
      | end
  Ground4 : Ground  InitFcn=|
      | try
      |    MBDS_BlockCallback('Update', gcb);
      | end
  Ground5 : Ground  InitFcn=|
      | try
      |    MBDS_BlockCallback('Update', gcb);
      | end
  Ground6 : Ground  InitFcn=|
      | try
      |    MBDS_BlockCallback('Update', gcb);
      | end
  Ground7 : Ground  InitFcn=|
      | try
      |    MBDS_BlockCallback('Update', gcb);
      | end
  Ground8 : Ground  InitFcn=|
      | try
      |    MBDS_BlockCallback('Update', gcb);
      | end
  Ground9 : Ground  InitFcn=|
      | try
      |    MBDS_BlockCallback('Update', gcb);
      | end
  L4_Controller : Subsystem  AncestorBlock=SUB_ECU_L4_MABX/L4_Controller
  Terminator : Terminator
  Out1 : Outport
  wires:
  L4_Controller/1(OUTPUTS) -> Out1/1
  input/1 -> Bus Selector/1
  Bus Selector/3 -> L4_Controller/3(BrakeSwitch)  "<SPN597_BrakeSwitch>"
  Bus Selector/4 -> L4_Controller/4(EBC2_FrontAxleSpeed)  "<SPN904_FrontAxleSpd>"
  Bus Selector/8 -> L4_Controller/8(SPN524_TransSelectedGear)  "<SPN524_TransSelectedGear>"
  Bus Selector/9 -> L4_Controller/9(SPN523_TransCurrentGear)  "<SPN523_TransCurrentGear>"
  Bus Selector/10 -> L4_Controller/10(SPN526_TransActGearRatio)  "<SPN526_TransActualGearRatio>"
  Bus Selector/11 -> L4_Controller/11(ActEngPercentTorque)  "<SPN513_ActualEngPercTorque>"
  Bus Selector/12 -> L4_Controller/12(ActEngPercentTorqueHightRes)  "<SPN4154_ActualEngPercTorqueFractional>"
  Bus Selector/13 -> L4_Controller/13(EngineSpeed)  "<SPN190_EngineSpeed>"
  Bus Selector/15 -> L4_Controller/15(SPN514_NominalFrictionPerTrq)  "<SPN514_NominalFrictionPercTorque>"
  Bus Selector/17 -> L4_Controller/17(SPN1760_GrossCombinationVehicleWeight)  "<SPN1760_GrossCombinationVehicleWeight>"
  L4_Controller/2(INPUTS1) -> Terminator/1
  Bus Selector/1 -> L4_Controller/1(OperatorEnableSwitch)  "<OperatorEnable>"
  Bus Selector/7 -> L4_Controller/7(EBSBrakeSwitch)  "<SPN1121_EBS_BrakeSwitch>"
  Bus Selector/16 -> L4_Controller/16(SPN2978_EstEngParasiticLossesPerTrq)  "<SPN2978_EstimatedEngineParasiticLossesPercTrq>"
  Bus Selector/20 -> L4_Controller/20(SPN544_EngineReferenceTorque)  "<SPN544_EngineReferenceTrq>"
  Bus Selector/21 -> L4_Controller/21(SPN1816_ROP_EngineControlActive)  "<SPN1816_ROP_EngineControlActive>"
  Bus Selector/22 -> L4_Controller/22(SPN1818_ROP_BrakeControlActive)  "<SPN1818_ROP_BrakeControlActive>"
  Bus Selector/23 -> L4_Controller/23(SPN1817_YC_EngineControlActive)  "<SPN1817_YC_EngineControlActive>"
  Bus Selector/24 -> L4_Controller/24(SPN1819_YC_BrakeControlActive)  "<SPN1819_YC_BrakeControlActive>"
  Bus Selector/25 -> L4_Controller/25(SteeringWheelAngle)  "<SPN1807_SteeringWheelAngle>"
  Bus Selector/26 -> L4_Controller/26(YawRate)  "<SPN1808_YawRate>"
  Constant/1 -> L4_Controller/34(PX2_LanePosEstPosition)
  Constant1/1 -> L4_Controller/35(PX2_LanePosEstAngle)
  Constant2/1 -> L4_Controller/36(PX2_LanePosEstNumPoints)
  Bus Selector/27 -> L4_Controller/27(SPN108_BarometricPressure)  "<SPN108_BarometricPressure>"
  Bus Selector/28 -> L4_Controller/28(SPN171_AmbientAirTemperature)  "<SPN171_AmbientAirTemperature>"
  Constant3/1 -> L4_Controller/29(VI_Truck1571VinMatch)
  Constant4/1 -> L4_Controller/30(SSI2_PitchAngleExtRange)
  Bus Selector/2 -> L4_Controller/2(PedalPWMPos)  "<PedDrv>"
  Bus Selector/5 -> L4_Controller/5(HRW_FrontAxleLeftWheelSpeed)  "<SPN1592_FrontAxleLeftWheelSpeed>"
  Bus Selector/6 -> L4_Controller/6(HRW_FrontAxleRightWheelSpeed)  "<SPN1593_FrontAxleRightWheelSpeed>"
  Bus Selector/29 -> L4_Controller/31(Latitude)  "<Latitude>"
  Bus Selector/30 -> L4_Controller/32(Longitude)  "<Longitude>"
  Bus Selector/31 -> L4_Controller/33(HDOP)  "<HDOP>"
  Bus Selector/18 -> L4_Controller/18(SPN1796_DistanceAlertSignal)  "<SPN1796_ACC_DistanceAlertSignal>"
  Bus Selector/19 -> L4_Controller/19(SPN5022_ForwardCollisionWarning)  "<SPN5022_ForwardCollisionWarning>"
  Bus Selector/14 -> L4_Controller/14(SPN512_DriversDemandEngPercentTorque)  "<SPN512_DriverDemandPercentTorque>"
  Constant5/1 -> L4_Controller/37(VI_Truck166VinMatch)
  Bus Selector/32 -> L4_Controller/38(SPN1810_LongitudinalAcceleration)  "<SPN1810_LongitudinalAcceleration>"
  Bus Selector/34 -> L4_Controller/40(SPN1812_SteeringWheelAngleSensorType)  "<SPN1812_SteeringWheelAngleSensorType>"
  Bus Selector/36 -> L4_Controller/42(<PIC_Bus>)  "<PIC_Bus>"
  Ground/1 -> L4_Controller/45(PressureP1)
  Ground1/1 -> L4_Controller/46(PressureP4)
  Ground2/1 -> L4_Controller/47(PressureP21)
  Ground3/1 -> L4_Controller/48(PressureP22)
  Ground4/1 -> L4_Controller/49(PressureP42)
  Ground5/1 -> L4_Controller/43(XPRControlMode)
  Ground7/1 -> L4_Controller/50(IgnitionKeySwitch_voltage)  "IgnitionKeySwitch_voltage"
  Ground8/1 -> L4_Controller/51(Park_brake_switch)  "Park_brake_switch"
  Ground6/1 -> L4_Controller/52(Cruise_control_enable_switch)  "Cruise_control_enable_switch"
  Bus Selector/35 -> L4_Controller/41(SPN1809_LateralAcceleration)  "<SPN1809_LateralAcceleration>"
  Bus Selector/33 -> L4_Controller/39(SPN1811_SteeringWheelTurnCounter)  "<SPN1811_SteeringWheelTurnCounter>"
  Ground9/1 -> L4_Controller/44(XPRErrorState)

== system L4_SIM/Controllers/Virtual_Controllers/PACC ==
  In1 : Inport
  Bus Creator : BusCreator  Inputs=1
  Bus Selector : BusSelector  OutputSignals=Feedback_controllers.PCI.CCData.CCSetSpdDrv
  Signal Conversion : SignalConversion  OverrideOpt=off
  Out1 : Outport
  wires:
  In1/1 -> Bus Selector/1
  Bus Creator/1 -> Out1/1
  Bus Selector/1 -> Signal Conversion/1  "<CCSetSpdDrv>"
  Signal Conversion/1 -> Bus Creator/1  "PACC_CCSetSpdAdj"

== system L4_SIM/Controllers/Virtual_Controllers/PCC ==
  In1 : Inport
  Bus Creator : BusCreator  Inputs=3
  SPN7316_PCC_SET_SPEED_OFFSET : Constant  Value=single(0)
  SPN7317_PCC_STATE : Constant  Value=ENUM_J1939_PCC_STATE_T.DISABLED
  SPN7430_PCC_DRIVELINE_DISENGAGE_INHIBIT : Constant  Value=ENUM_J1939_SWITCH_T.OFF
  Terminator : Terminator
      settings: InitFcn=|
      | try
      |    MBDS_BlockCallback('Update', gcb);
      | end
  Out1 : Outport
  wires:
  In1/1 -> Terminator/1
  Bus Creator/1 -> Out1/1  "PCC"
  SPN7316_PCC_SET_SPEED_OFFSET/1 -> Bus Creator/1  "PCCSetSpeedOffset"
  SPN7317_PCC_STATE/1 -> Bus Creator/2  "PCCState"
  SPN7430_PCC_DRIVELINE_DISENGAGE_INHIBIT/1 -> Bus Creator/3  "PCCDrivelineDisengageInhibit"

== system L4_SIM/Controllers/Virtual_Controllers/PCI ==
  In : Inport
  Bus Creator : BusCreator  Inputs=5
  Bus Creator1 : BusCreator  Inputs=11
  Bus Selector : BusSelector  OutputSignals=CAN.CCVS1_00.SPN86_CruiseControlSetSpeed,CAN.CCVS1_00.SPN84_WheelBasedVehicleSpeed,CAN.PCC1_4B.SPN7316_PCCSetSpeedOffset,CAN.ETC1_00.SPN560_TransDrivelineEngaged,CAN.ACC1_2A.SPN1586_SpeedOfForwardVehicle,CAN.ETC2_00.SPN526_TransActualGearRatio,CAN.CVW_0B.SPN1760_GrossCombinationVehicleWeight
  Bus Selector1 : BusSelector  OutputSignals=Feedback_controllers.ABS.TSC1_P32_BR,Feedback_controllers.AMT.ShiftControl.External.TSC1_P32_TR,Feedback_controllers.VEMC.TSC1_P32_VEMCR
  Bus Selector2 : BusSelector  OutputSignals=Operator.PedDrv,Feedback_controllers.ABS.TSC1_P32_BE,Feedback_controllers.AMT.ShiftControl.External.TSC1_P32_TE,Feedback_controllers.VECU.TSC1_P4_VECU,Feedback_controllers.VEMC.TSC1_P2_VEMCE,Feedback_controllers.ERAD.TSC1_P5_ERAD
  Bus Selector3 : BusSelector  OutputSignals=CAN.CCVS1_00.SPN84_WheelBasedVehicleSpeed
  Constant3 : PTC_MBDS_LIB/Extras/Sources/Constant  Value2=true  PTC_MBDS_BlockVersion=5.41  PTC_BlockType=PTC_MBDS_Constant
      settings: SourceProductName=PACCAR Technical Center MBDS Library
  CruiseController : SUB_ECU_CruiseController/CruiseController
  Gain1 : Gain  Gain=100
  Gain2 : Gain  Gain=100
  Mux : Mux  Inputs=3
  Mux1 : Mux  Inputs=2
  Mux2 : Mux  Inputs=2
  Scope : Scope  NumInputPorts=3
  Scope1 : Scope  NumInputPorts=2
  Signal Conversion : SignalConversion  OverrideOpt=off
  TSC Engine Arbitration : Subsystem
  TSC Retarder Arbitration : Subsystem
  Terminator : Terminator
  Out1 : Outport
  wires:
  CruiseController/4 -> Bus Creator1/2
  CruiseController/5 -> Bus Creator1/3
  CruiseController/6 -> Bus Creator1/4
  CruiseController/7 -> Mux/1, Bus Creator1/5
  CruiseController/8 -> Bus Creator1/6
  CruiseController/9 -> Mux/2, Bus Creator1/7
  CruiseController/10 -> Bus Creator1/8
  CruiseController/12 -> Bus Creator1/10
  CruiseController/11 -> Bus Creator1/9
  Constant3/1 -> CruiseController/Enable
  CruiseController/1 -> Scope/2, [CrsTrqDem]
  Mux/1 -> Scope/1
  CruiseController/3 -> Bus Creator1/1
  Gain2/1 -> Mux1/2
  Bus Selector/5 -> CruiseController/5  "<SPN1586_SpeedOfForwardVehicle>"
  In/1 -> Bus Selector3/1, Bus Selector2/1, Bus Selector1/1, Bus Selector/1
  Mux2/1 -> Scope1/2
  Gain1/1 -> Mux2/2
  Bus Selector2/4 -> TSC Engine Arbitration/5(TSC1_P4_VECU)  "<TSC1_P4_VECU>"
  Bus Selector2/2 -> TSC Engine Arbitration/3(TSC1_P32_BE)  "<TSC1_P32_BE>"
  Bus Selector1/3 -> TSC Retarder Arbitration/4(TSC1_P32_VEMCR)  "<TSC1_P32_VEMCR>"
  [CrsTrqDem] -> TSC Engine Arbitration/1(CrsTrqDem)
  Bus Selector2/6 -> TSC Engine Arbitration/7(TSC1_P5_ERAD)  "<TSC1_P5_ERAD>"
  Bus Selector2/3 -> TSC Engine Arbitration/4(TSC1_P32_TE)  "<TSC1_P32_TE>"
  Bus Selector/3 -> CruiseController/3  "<SPN7316_PCCSetSpeedOffset>"
  Bus Selector2/1 -> TSC Engine Arbitration/2(PedDvr)  "<PedDrv>"
  TSC Engine Arbitration/1(DriverDemPercentTrq) -> Mux1/1, Bus Creator/3
  TSC Engine Arbitration/2(EngTrqDemand) -> Gain2/1, Bus Creator/4
  Bus Selector1/1 -> TSC Retarder Arbitration/2(TSC1_P32_BR)  "<TSC1_P32_BR>"
  Mux1/1 -> Scope1/1
  Bus Selector/7 -> CruiseController/7  "<SPN1760_GrossCombinationVehicleWeight>"
  Bus Selector/6 -> CruiseController/6  "<SPN526_TransActualGearRatio>"
  Bus Selector/2 -> Mux/3, CruiseController/2  "<SPN84_WheelBasedVehicleSpeed>"
  Bus Selector1/2 -> TSC Retarder Arbitration/3(TSC1_P32_TR)  "<TSC1_P32_TR>"
  Bus Selector/4 -> CruiseController/4  "<SPN560_TransDrivelineEngaged>"
  Bus Selector2/5 -> TSC Engine Arbitration/6(TSC1_P2_VEMCE)  "<TSC1_P2_VEMCE>"
  Bus Selector/1 -> CruiseController/1  "<SPN86_CruiseControlSetSpeed>"
  Bus Creator1/1 -> Bus Creator/1  "CCData"
  TSC Retarder Arbitration/1(DriverDemandRetarderPercentTorque) -> Mux2/1, Bus Creator1/11
  TSC Retarder Arbitration/2(EngRetarderDemand) -> Bus Creator/2, Gain1/1
  Bus Creator/1 -> Out1/1
  CruiseController/2 -> [CrsRetDem], Scope/3
  [CrsRetDem] -> TSC Retarder Arbitration/1(CrsRetDem)
  CruiseController/13 -> Terminator/1
  Bus Selector3/1 -> Signal Conversion/1  "<SPN84_WheelBasedVehicleSpeed>"
  Signal Conversion/1 -> Bus Creator/5  "EngSpeedRPM"

== system L4_SIM/Controllers/Virtual_Controllers/TCM ==
  In1 : Inport
  Bus Creator : BusCreator  Inputs=1
  Bus Creator1 : BusCreator  Inputs=8
  Bus Creator3 : BusCreator  Inputs=2
  Bus Creator4 : BusCreator  Inputs=5
  Bus Selector : BusSelector  OutputSignals=TrqReqE
  Bus Selector1 : BusSelector  OutputSignals=TrqReqR
  Bus Selector3 : BusSelector  OutputSignals=CoastCtrlState,CoastVehAccelCond,CoastVehVBrkAct,CoastVehSpdCond
  Bus Selector4 : BusSelector  OutputSignals=CAN.EBC1_0B.SPN521_BrakePedalPosition,CAN.ERC1_0F.SPN1715_DriverDemandRetarderPercentTorque,CAN.CVW_0B.SPN1760_GrossCombinationVehicleWeight,CAN.SSI2_03.SPN4976_PitchAngleExtendedRange,CAN.ERC1_0F.SPN520_ActualRetarderPercentTorque,CAN.EEC1_00.SPN190_EngineSpeed,CAN.EEC1_00.SPN513_ActualEngPercTorque,CAN.EEC3_00.SPN514_NominalFrictionPercTorque,CAN.EEC1_00.SPN512_DriverDemandPercentTorque,Feedback_controllers.PACC.PACC_CCSetSpdAdj,Feedback_controllers.VEMC.NeutralCoastRequest,Feedback_sensors.Chassis.VehAccel,CAN.CCVS1_00.SPN84_WheelBasedVehicleSpeed,Feedback_sensors.Chassis.GearNumber,Feedback_sensors.Chassis.TransmissionStateLock
  Gain1 : Gain  Gain=0.01
  Gain2 : Gain  Gain=0.01
  Logical Operator1 : Logic  Operator=NOT  AllPortsSameDT=off  OutDataTypeStr=boolean
  Mux : Mux  Inputs=2
  Mux1 : Mux  Inputs=2
  Mux2 : Mux  Inputs=2
  Scope : Scope  NumInputPorts=5
  SignalConversion1 : SignalConversion  ConversionOutput=Contiguous copy  OverrideOpt=off
  SignalConversion2 : SignalConversion  ConversionOutput=Contiguous copy  OverrideOpt=off
  SignalConversion3 : SignalConversion  ConversionOutput=Contiguous copy  OverrideOpt=off
  TCM : SUB_ECU_Transmission/TCM
  Out1 : Outport
  wires:
  Bus Creator/1 -> Out1/1
  Bus Selector4/12 -> TCM/12  "<VehAccel>"
  Bus Selector4/15 -> TCM/15, SignalConversion1/1  "<TransmissionStateLock>"
  Bus Selector4/4 -> TCM/4  "<SPN4976_PitchAngleExtendedRange>"
  Bus Selector4/14 -> TCM/14, SignalConversion2/1  "<GearNumber>"
  Bus Creator4/1 -> Bus Creator3/2  "External"
  Bus Creator1/1 -> Bus Creator3/1  "Internal"
  Bus Creator3/1 -> Bus Creator/1  "ShiftControl"
  SignalConversion1/1 -> Bus Creator4/5  "TransStateLock"
  SignalConversion2/1 -> Bus Creator4/4  "GearNumberActual"
  Bus Selector3/3 -> Bus Creator1/3  "<CoastVehVBrkAct>"
  Bus Selector3/2 -> Bus Creator1/2  "<CoastVehAccelCond>"
  Bus Selector3/4 -> Bus Creator1/4  "<CoastVehSpdCond>"
  Bus Selector3/1 -> Bus Creator1/1  "<CoastCtrlState>"
  TCM/1 -> Bus Selector3/1
  TCM/6 -> Bus Creator4/2, Bus Selector/1
  TCM/7 -> Bus Creator4/3, Bus Selector1/1
  In1/1 -> Bus Selector4/1
  Bus Selector4/1 -> TCM/1  "<SPN521_BrakePedalPosition>"
  Bus Selector4/2 -> TCM/2, Gain2/1  "<SPN1715_DriverDemandRetarderPercentTorque>"
  Bus Selector4/3 -> TCM/3  "<SPN1760_GrossCombinationVehicleWeight>"
  Bus Selector4/5 -> TCM/5  "<SPN520_ActualRetarderPercentTorque>"
  Bus Selector4/6 -> TCM/6  "<SPN190_EngineSpeed>"
  Bus Selector4/7 -> TCM/7  "<SPN513_ActualEngPercTorque>"
  Bus Selector4/8 -> TCM/8  "<SPN514_NominalFrictionPercTorque>"
  Bus Selector4/9 -> TCM/9, Gain1/1  "<SPN512_DriverDemandPercentTorque>"
  Bus Selector4/11 -> TCM/11  "<NeutralCoastRequest>"
  SignalConversion3/1 -> Bus Creator4/1  "GearNumberRequest"
  Bus Selector4/10 -> TCM/10  "<PACC_CCSetSpdAdj>"
  Mux2/1 -> Scope/3
  Mux1/1 -> Scope/1
  Mux/1 -> Scope/2
  TCM/4 -> Bus Creator1/7, Scope/4
  Gain2/1 -> Mux2/1
  Gain1/1 -> Mux/1
  TCM/3 -> Bus Creator1/6, Logical Operator1/1
  Logical Operator1/1 -> Mux1/2
  TCM/5 -> Scope/5, SignalConversion3/1, Bus Creator1/8
  TCM/2 -> Bus Creator1/5, Mux1/1
  Bus Selector1/1 -> Mux2/2  "<TrqReqR>"
  Bus Selector/1 -> Mux/2  "<TrqReqE>"
  Bus Selector4/13 -> TCM/13  "<SPN84_WheelBasedVehicleSpeed>"
